simulink model "exam4"  (R2016a)
settings: Solver=VariableStepAuto  StartTime=0.0  StopTime=10.0  RelTol=1e-3
settings Model: Creator=linghao  LastModifiedBy=linghao
settings GRTTargetCC: GeneratePreprocessorConditionals=Use local settings

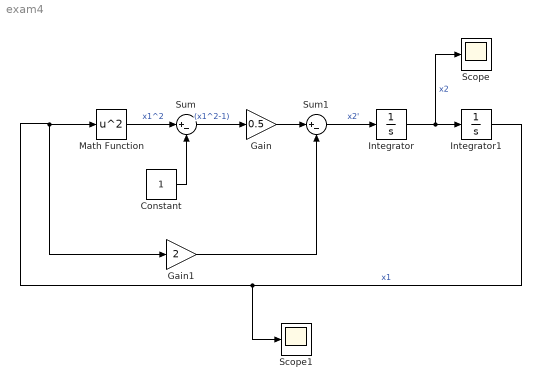
== system exam4 ==
  Constant : Constant
  Gain : Gain  Gain=0.5
  Gain1 : Gain  Gain=2
  Integrator : Integrator  InitialCondition=2
  Integrator1 : Integrator  InitialCondition=-1
  Math Function : Math  Operator=square  SaturateOnIntegerOverflow=on
  Scope : Scope
  Scope1 : Scope
  Sum : Sum  Inputs=|+-
  Sum1 : Sum  Inputs=|+-
  wires:
  Sum/1 -> Gain/1  "(x1^2-1)"
  Constant/1 -> Sum/2
  Math Function/1 -> Sum/1  "x1^2"
  Gain/1 -> Sum1/1
  Integrator1/1 -> Scope1/1, Gain1/1, Math Function/1  "x1"
  Gain1/1 -> Sum1/2
  Sum1/1 -> Integrator/1  "x2'"
  Integrator/1 -> Scope/1, Integrator1/1  "x2"
